simulink model "Tram_control_scheme"  (R2021a)
settings: Solver=VariableStepAuto  StartTime=0.0  StopTime=2000
values from neighbouring files (symbols this model uses):
  B = Tfriction/rated_speed_motor    (= 0.814101549937)    [Tram_script.m]
  d = 680e-3    (= 0.68)    [Tram_script.m]
  distance = [0,1,1.001,3,3.001,4,4.001,6,6.001,8,8.001,9,9.001,10]    [Tram_script.m]
  E = Van-Ra*Ian    (= 540)    [Tram_script.m]
  Ian = Pel_eq/Van    (= 155.555555556)    [Tram_script.m]
  Ien = 5    [Tram_script.m]
  J_eq = m_full_load*((speed_tram/3.6)^2)/(rated_speed_motor^2)    (= 85.9801387874)    [Tram_script.m]
  K = Tn/(Ian*Ien)    (= 1.06322065076)    [Tram_script.m]
  ki_a = par_regi.Ki    [Tram_script.m]
  ki_e = par_rege.Ki    [Tram_script.m]
  ki_O = par_reg_speed.Ki    [Tram_script.m]
  kp_a = par_regi.Kp    [Tram_script.m]
  kp_e = par_rege.Kp    [Tram_script.m]
  kp_O = par_reg_speed.Kp    [Tram_script.m]
  La = tau_a*Ra    (= 0.00385714285714)    [Tram_script.m]
  Le = Re*tau_e    (= 1.2)    [Tram_script.m]
  Ra = (1-efficiency)*Van/Ian    (= 0.385714285714)    [Tram_script.m]
  rated_speed_motor = Or*(2*pi)/60    (= 101.578162466)    [Tram_script.m]
  Re = Ven/Ien    (= 12)    [Tram_script.m]
  rho = 13/74    (= 0.175675675676)    [Tram_script.m]
  SatLow_T = -Tn*3    (= -2480.8481851)    [Tram_script.m]
  SatLow_Va = -Van    (= -600)    [Tram_script.m]
  SatLow_Ve = 0    [Tram_script.m]
  SatUp_T = Tn*3    (= 2480.8481851)    [Tram_script.m]
  SatUp_Va = Van    (= 600)    [Tram_script.m]
  SatUp_Ve = Ven*1.1    (= 66)    [Tram_script.m]
  speed_ref = [speed_tram/2,speed_tram/2, speed_tram,speed_tram,speed_tram,speed_tram,speed_max,speed_max,speed_tram,speed_tram,speed_tram,speed_tram,speed_tram/2,speed_tram/2]    [Tram_script.m]
  speed_weak = [0, speed_tram/4,speed_tram/2, speed_tram,speed_tram*1.5, speed_tram*1.8,speed_tram*1.9 speed_tram*2]    [Tram_script.m]
  T_weakening = [Tn, Tn, Tn, Tn, Tn/1.5, Tn/2, Tn/2.5, Tn/5]    [Tram_script.m]
  Tfriction = Tn/10    (= 82.6949395034)    [Tram_script.m]
  Ti_a = kp_a/ki_a    [Tram_script.m]
  Ti_e = kp_e/ki_e    [Tram_script.m]
  Ti_O = kp_O/ki_O    [Tram_script.m]
  Tn = Pmec_eq/rated_speed_motor    (= 826.949395034)    [Tram_script.m]
  Tslope = m_full_load*9.81*sin(theta)*d/2*rho    [Tram_script.m]
libraries: pid_lib x3, simulink x2, spspowerguiLib x1
settings Model: Creator=secch  LastModifiedBy=secch
settings SolverCC: AlgebraicLoopSolver=LineSearch
settings DebuggingCC: SFMachineParentedDataDiag=warning

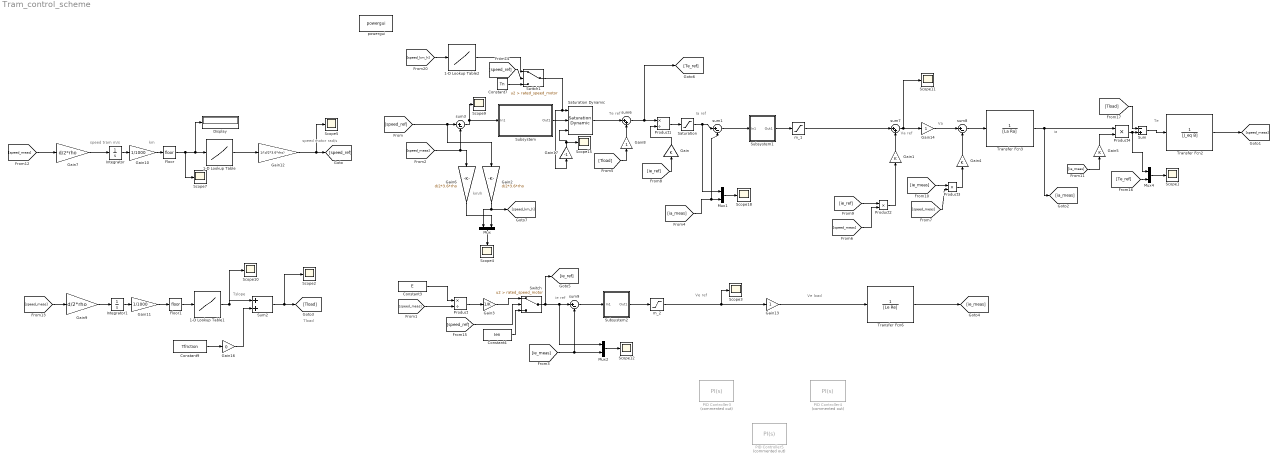
== system Tram_control_scheme ==
  note: km/h
  note: km
  note: speed tram
      | m/s
  note: speed motor
      | rad/s
  note: ia
  note: Va ref
  note: Ve load
  note: ie ref
  note: Te
  note: Ia ref
  note: Te ref
  note: Tload
  note: Tslope
  note: Ve ref
  note: Va
  1-D Lookup Table : Lookup_n-D  NumberOfTableDimensions=1  BreakpointsForDimension1=distance  Table=speed_ref  InternalRulePriority=Speed  RndMeth=Simplest  InputSameDT=on
  1-D Lookup Table1 : Lookup_n-D  NumberOfTableDimensions=1  BreakpointsForDimension1=distance  Table=Tslope  InternalRulePriority=Speed  RndMeth=Simplest  InputSameDT=on
  1-D Lookup Table2 : Lookup_n-D  NumberOfTableDimensions=1  BreakpointsForDimension1=speed_weak  Table=T_weakening  InternalRulePriority=Speed  RndMeth=Simplest  InputSameDT=on
  Constant3 : Constant  Value=E
  Constant4 : Constant  Value=Ien
  Constant7 : Constant  Value=Tn
  Constant9 : Constant  Value=Tfriction
  Display : Display
  Floor : Rounding
  Floor1 : Rounding
  Gain{,1,4..5} (4 alike) : Gain  Gain=K
  Gain10 : Gain  Gain=1/1000
  Gain11 : Gain  Gain=1/1000
  Gain12 : Gain  Gain=1/(d/2*3.6*rho)
  Gain13 : Gain
  Gain14 : Gain
  Gain16 : Gain  Gain=0
  Gain17 : Gain  Gain=-1
  Gain2 : Gain  Gain=d/2*3.6*rho
  Gain3 : Gain  Gain=1/K
  Gain6 : Gain  Gain=d/2*3.6*rho
  Gain7 : Gain  Gain=d/2*rho
  Gain8 : Gain
  Gain9 : Gain  Gain=d/2*rho
  Integrator : Integrator
  Integrator1 : Integrator
  Mux{,1..2,4} (4 alike) : Mux  Inputs=2
  PID Controller3 : pid_lib/PID Controller  Commented=on  Controller=PI  Form=Ideal  TimeDomain=Continuous-time  UseExternalTs=off  SampleTime=-1  IntegratorMethod=Forward Euler  FilterMethod=Forward Euler  ControllerParametersSource=internal  P=kp_O  I=ki_O  D=0  UseFilter=on  N=100  TunerSelectOption=Transfer Function Based (PID Tuner App)  InitialConditionSource=internal  InitialConditionForIntegrator=0  InitialConditionForFilter=0  DifferentiatorICPrevScaledInput=0  ExternalReset=none  TrackingMode=off  Kt=1  LimitOutput=on  SatLimitsSource=internal  UpperSaturationLimit=SatUp_T  LowerSaturationLimit=SatLow_T  LinearizeAsGain=on  AntiWindupMode=back-calculation  Kb=Ti_O  POutMin=[]  POutMax=[]  IOutMin=[]  IOutMax=[]  DOutMin=[]  DOutMax=[]  NOutMin=[]  NOutMax=[]  SumOutMin=[]  SumOutMax=[]  SaturationOutMin=[]  SaturationOutMax=[]  PParamMin=[]  PParamMax=[]  IParamMin=[]  IParamMax=[]  DParamMin=[]  DParamMax=[]  NParamMin=[]  NParamMax=[]  KbParamMin=[]  KbParamMax=[]  KtParamMin=[]  KtParamMax=[]  KbOutMin=[]  KbOutMax=[]  KtOutMin=[]  KtOutMax=[]  IntegratorOutMin=[]  IntegratorOutMax=[]  FilterOutMin=[]  FilterOutMax=[]  SumI1OutMin=[]  SumI1OutMax=[]  SumI2OutMin=[]  SumI2OutMax=[]  SumI3OutMin=[]  SumI3OutMax=[]  SumI4OutMin=[]  SumI4OutMax=[]  SumDOutMin=[]  SumDOutMax=[]  DifferentiatorOutMin=[]  DifferentiatorOutMax=[]  FilterDiffOutCoefMin=[]  FilterDiffOutCoefMax=[]  ReciprocalOutMin=[]  ReciprocalOutMax=[]  SumDenOutMin=[]  SumDenOutMax=[]  SumNumOutMin=[]  SumNumOutMax=[]  DivideOutMin=[]  DivideOutMax=[]  UdiffTsProdOutMin=[]  UdiffTsProdOutMax=[]  NTsProdOutMin=[]  NTsProdOutMax=[]  UintegralTsProdOutMin=[]  UintegralTsProdOutMax=[]  UngainTsProdOutMin=[]  UngainTsProdOutMax=[]  IntegratorContinuousStateAttributes=''  IntegratorStateMustResolveToSignalObject=off  IntegratorRTWStateStorageClass=Auto  FilterContinuousStateAttributes=''  FilterStateMustResolveToSignalObject=off  FilterRTWStateStorageClass=Auto  ParallelPVariant=Passthrough  IdealPVariant=InternalParameters  IVariant=InternalParameters  DVariant=Disabled  IntegratorVariant=Continuous  SatVariant=Enabled  AWVariant=BackCalculation  PCopyVariant=Disabled  TRVariant=Disabled  FdbkBlocksVariant=Forward  IdealPFdbkVariant=Disabled  SatFdbkVariant=Disabled  DerivativeFilterVariant=Disabled  NVariant=Disabled  NCopyVariant=Disabled_SignalSpec  FilterICVariant=Disabled  IntegratorICVariant=InternalICs  ExternalResetVariant=Disabled  TRSumVariant=Passthrough  SumFdbkVariant=Disabled  SumVariant=Sum_PI  TsampFilterVariant=InternalTs  TsampNgainVariant=Passthrough  TsampIntegralVariant=Passthrough  ExternalSaturationOutDataTypeStr=Inherit: Same as second input
  PID Controller4 : pid_lib/PID Controller  Commented=on  Controller=PI  Form=Ideal  TimeDomain=Continuous-time  UseExternalTs=off  SampleTime=-1  IntegratorMethod=Forward Euler  FilterMethod=Forward Euler  ControllerParametersSource=internal  P=kp_a  I=ki_a  D=0  UseFilter=on  N=100  TunerSelectOption=Transfer Function Based (PID Tuner App)  InitialConditionSource=internal  InitialConditionForIntegrator=0  InitialConditionForFilter=0  DifferentiatorICPrevScaledInput=0  ExternalReset=none  TrackingMode=off  Kt=1  LimitOutput=on  SatLimitsSource=internal  UpperSaturationLimit=SatUp_Va  LowerSaturationLimit=SatLow_Va  LinearizeAsGain=on  AntiWindupMode=back-calculation  Kb=Ti_a  POutMin=[]  POutMax=[]  IOutMin=[]  IOutMax=[]  DOutMin=[]  DOutMax=[]  NOutMin=[]  NOutMax=[]  SumOutMin=[]  SumOutMax=[]  SaturationOutMin=[]  SaturationOutMax=[]  PParamMin=[]  PParamMax=[]  IParamMin=[]  IParamMax=[]  DParamMin=[]  DParamMax=[]  NParamMin=[]  NParamMax=[]  KbParamMin=[]  KbParamMax=[]  KtParamMin=[]  KtParamMax=[]  KbOutMin=[]  KbOutMax=[]  KtOutMin=[]  KtOutMax=[]  IntegratorOutMin=[]  IntegratorOutMax=[]  FilterOutMin=[]  FilterOutMax=[]  SumI1OutMin=[]  SumI1OutMax=[]  SumI2OutMin=[]  SumI2OutMax=[]  SumI3OutMin=[]  SumI3OutMax=[]  SumI4OutMin=[]  SumI4OutMax=[]  SumDOutMin=[]  SumDOutMax=[]  DifferentiatorOutMin=[]  DifferentiatorOutMax=[]  FilterDiffOutCoefMin=[]  FilterDiffOutCoefMax=[]  ReciprocalOutMin=[]  ReciprocalOutMax=[]  SumDenOutMin=[]  SumDenOutMax=[]  SumNumOutMin=[]  SumNumOutMax=[]  DivideOutMin=[]  DivideOutMax=[]  UdiffTsProdOutMin=[]  UdiffTsProdOutMax=[]  NTsProdOutMin=[]  NTsProdOutMax=[]  UintegralTsProdOutMin=[]  UintegralTsProdOutMax=[]  UngainTsProdOutMin=[]  UngainTsProdOutMax=[]  IntegratorContinuousStateAttributes=''  IntegratorStateMustResolveToSignalObject=off  IntegratorRTWStateStorageClass=Auto  FilterContinuousStateAttributes=''  FilterStateMustResolveToSignalObject=off  FilterRTWStateStorageClass=Auto  ParallelPVariant=Passthrough  IdealPVariant=InternalParameters  IVariant=InternalParameters  DVariant=Disabled  IntegratorVariant=Continuous  SatVariant=Enabled  AWVariant=BackCalculation  PCopyVariant=Disabled  TRVariant=Disabled  FdbkBlocksVariant=Forward  IdealPFdbkVariant=Disabled  SatFdbkVariant=Disabled  DerivativeFilterVariant=Disabled  NVariant=Disabled  NCopyVariant=Disabled_SignalSpec  FilterICVariant=Disabled  IntegratorICVariant=InternalICs  ExternalResetVariant=Disabled  TRSumVariant=Passthrough  SumFdbkVariant=Disabled  SumVariant=Sum_PI  TsampFilterVariant=InternalTs  TsampNgainVariant=Passthrough  TsampIntegralVariant=Passthrough  ExternalSaturationOutDataTypeStr=Inherit: Same as second input
  PID Controller5 : pid_lib/PID Controller  Commented=on  Controller=PI  Form=Ideal  TimeDomain=Continuous-time  UseExternalTs=off  SampleTime=-1  IntegratorMethod=Forward Euler  FilterMethod=Forward Euler  ControllerParametersSource=internal  P=kp_e  I=ki_e  D=0  UseFilter=on  N=100  TunerSelectOption=Transfer Function Based (PID Tuner App)  InitialConditionSource=internal  InitialConditionForIntegrator=0  InitialConditionForFilter=0  DifferentiatorICPrevScaledInput=0  ExternalReset=none  TrackingMode=off  Kt=1  LimitOutput=on  SatLimitsSource=internal  UpperSaturationLimit=SatUp_Ve  LowerSaturationLimit=SatLow_Ve  LinearizeAsGain=on  AntiWindupMode=back-calculation  Kb=Ti_e  POutMin=[]  POutMax=[]  IOutMin=[]  IOutMax=[]  DOutMin=[]  DOutMax=[]  NOutMin=[]  NOutMax=[]  SumOutMin=[]  SumOutMax=[]  SaturationOutMin=[]  SaturationOutMax=[]  PParamMin=[]  PParamMax=[]  IParamMin=[]  IParamMax=[]  DParamMin=[]  DParamMax=[]  NParamMin=[]  NParamMax=[]  KbParamMin=[]  KbParamMax=[]  KtParamMin=[]  KtParamMax=[]  KbOutMin=[]  KbOutMax=[]  KtOutMin=[]  KtOutMax=[]  IntegratorOutMin=[]  IntegratorOutMax=[]  FilterOutMin=[]  FilterOutMax=[]  SumI1OutMin=[]  SumI1OutMax=[]  SumI2OutMin=[]  SumI2OutMax=[]  SumI3OutMin=[]  SumI3OutMax=[]  SumI4OutMin=[]  SumI4OutMax=[]  SumDOutMin=[]  SumDOutMax=[]  DifferentiatorOutMin=[]  DifferentiatorOutMax=[]  FilterDiffOutCoefMin=[]  FilterDiffOutCoefMax=[]  ReciprocalOutMin=[]  ReciprocalOutMax=[]  SumDenOutMin=[]  SumDenOutMax=[]  SumNumOutMin=[]  SumNumOutMax=[]  DivideOutMin=[]  DivideOutMax=[]  UdiffTsProdOutMin=[]  UdiffTsProdOutMax=[]  NTsProdOutMin=[]  NTsProdOutMax=[]  UintegralTsProdOutMin=[]  UintegralTsProdOutMax=[]  UngainTsProdOutMin=[]  UngainTsProdOutMax=[]  IntegratorContinuousStateAttributes=''  IntegratorStateMustResolveToSignalObject=off  IntegratorRTWStateStorageClass=Auto  FilterContinuousStateAttributes=''  FilterStateMustResolveToSignalObject=off  FilterRTWStateStorageClass=Auto  ParallelPVariant=Passthrough  IdealPVariant=InternalParameters  IVariant=InternalParameters  DVariant=Disabled  IntegratorVariant=Continuous  SatVariant=Enabled  AWVariant=BackCalculation  PCopyVariant=Disabled  TRVariant=Disabled  FdbkBlocksVariant=Forward  IdealPFdbkVariant=Disabled  SatFdbkVariant=Disabled  DerivativeFilterVariant=Disabled  NVariant=Disabled  NCopyVariant=Disabled_SignalSpec  FilterICVariant=Disabled  IntegratorICVariant=InternalICs  ExternalResetVariant=Disabled  TRSumVariant=Passthrough  SumFdbkVariant=Disabled  SumVariant=Sum_PI  TsampFilterVariant=InternalTs  TsampNgainVariant=Passthrough  TsampIntegralVariant=Passthrough  ExternalSaturationOutDataTypeStr=Inherit: Same as second input
  Product : Product  Inputs=*/
  Product1 : Product  Inputs=*/
  Product2 : Product
  Product3 : Product
  Product4 : Product
  Saturation : Saturate  UpperLimit=Ian  LowerLimit=-Ian
  Saturation Dynamic : simulink/Discontinuities/Saturation Dynamic  OutMin=[]  OutMax=[]  OutDataTypeStr=Inherit: Same as second input  OutDataType=fixdt(1, 16)  OutScaling=2^-10  DoSatur=off
  Scope{1..5,7,9..12,15,18} (12 alike) : Scope
  Subsystem : Subsystem
  Subsystem1 : Subsystem
  Subsystem2 : Subsystem
  Sum : Sum  Inputs=-+
  Sum2 : Sum  Inputs=|++
  Switch : Switch  Criteria=u2 > Threshold  Threshold=rated_speed_motor
  Switch1 : Switch  Criteria=u2 > Threshold  Threshold=rated_speed_motor
  Transfer Fcn2 : TransferFcn  Denominator=[J_eq B]
  Transfer Fcn3 : TransferFcn  Denominator=[La Ra]
  Transfer Fcn6 : TransferFcn  Denominator=[Le Re]
  m_1 : Saturate  UpperLimit=SatUp_Va  LowerLimit=SatLow_Va
  m_2 : Saturate  UpperLimit=SatUp_Ve  LowerLimit=SatLow_Ve
  powergui : spspowerguiLib/powergui  Priority=1  SimulationMode=Continuous  SampleTime=50e-6  frequency=60  Iterations=50  frequencyindice=0  Pbase=100e6  ErrMax=1e-4  UnitsV=kV  UnitsW=MW  buscounter=0  FunctionMessages=off  echomessages=off  EnableUseOfTLC=off  CurrentSourceSwitches=off  DisableSnubberDevices=off  DisableRonSwitches=off  DisableVfSwitches=off  DisplayEquations=off  AutomaticDiscreteSolvers=off  SolverType=Tustin/Backward Euler (TBE)  Interpol=off  ExternalGateDelay=off  methode=off  Ts=100  x0status=blocks  SPID=on  SwTol=0  HookPort=off  NonlinearTolerance=1e-4  nMaxIteration=100  ContinueOnMaxIteration=off  RestoreLinks=warning  ResistiveCurrentMeasurement=off  Frange=[0:2:500]  Ylog=off  Xlog=on  ShowGrid=off  save=off  variable=ZData  structure=0  ZoomFFT=off  StartTime=0.0  cycles=1  DisplayStyle=1  fundamental=60  FreqAxis=off  MaxFrequency=1000  frequencyindicesteady=1  RmsSteady=1  display=off
  sum{1,3,8..9} (4 alike) : Sum  Inputs=|+-
  sum6 : Sum  Inputs=|++
  sum7 : Sum  Inputs=|++
  wires:
  sum3/1 -> Subsystem/1(In1), Scope9/1
  [speed_ref] -> Gain2/1, sum3/1
  Product1/1 -> Saturation/1
  sum8/1 -> Transfer Fcn3/1
  Transfer Fcn3/1 -> [ia_meas], Product4/1
  Product4/1 -> Mux4/1, Sum/2
  Constant3/1 -> Product/1
  Gain3/1 -> Switch/1
  Product/1 -> Gain3/1
  Constant4/1 -> Switch/3
  1-D Lookup Table1/1 -> Scope10/1, Sum2/1
  Constant9/1 -> Gain16/1
  [speed_meas] -> sum3/2, Gain6/1
  Transfer Fcn2/1 -> [speed_meas]
  [ie_ref] -> Gain/1
  [ia_meas] -> Mux1/2, sum1/2
  Product3/1 -> Gain4/1
  Sum2/1 -> Scope2/1, [Tload]
  [Tload] -> Gain8/1
  [ie_ref] -> Product2/1
  Product2/1 -> Gain1/1
  [speed_meas] -> Product2/2
  [speed_meas] -> Product3/2
  [ie_meas] -> Product3/1
  Switch/1 -> [ie_ref], Mux2/1, sum9/1
  [ie_meas] -> Mux2/2, sum9/2
  Gain13/1 -> Transfer Fcn6/1
  Transfer Fcn6/1 -> [ie_meas]
  sum7/1 -> Gain14/1, Scope11/1
  Gain14/1 -> sum8/1
  [ie_meas] -> Gain5/1
  Gain/1 -> Product1/2
  Gain1/1 -> sum7/2
  Gain4/1 -> sum8/2
  Gain5/1 -> Product4/2
  Gain7/1 -> Integrator/1
  Integrator/1 -> Gain10/1
  Floor/1 -> Scope7/1, 1-D Lookup Table/1, Display/1
  Floor1/1 -> 1-D Lookup Table1/1
  Integrator1/1 -> Gain11/1
  [speed_meas] -> Gain9/1
  Gain9/1 -> Integrator1/1
  sum6/1 -> [Te_ref], Product1/1
  Mux/1 -> Scope4/1
  Gain10/1 -> Floor/1
  [speed_meas] -> Product/2
  Gain11/1 -> Floor1/1
  [speed_ref] -> Switch/2
  Subsystem1/1(Out1) -> m_1/1
  sum1/1 -> Subsystem1/1(In1)
  Subsystem2/1(Out1) -> m_2/1
  sum9/1 -> Subsystem2/1(In1)
  Gain2/1 -> [speed_km_h], Mux/1
  Gain6/1 -> Mux/2
  [speed_meas] -> Gain7/1
  [speed_ref] -> Switch1/2
  Constant7/1 -> Switch1/3
  Gain17/1 -> Saturation Dynamic/3, Scope15/1
  Subsystem/1(Out1) -> Saturation Dynamic/2
  Saturation Dynamic/1 -> sum6/1
  m_1/1 -> sum7/1
  m_2/1 -> Gain13/1, Scope3/1
  Mux1/1 -> Scope18/1
  Mux2/1 -> Scope12/1
  Gain12/1 -> Scope5/1, [speed_ref]
  1-D Lookup Table/1 -> Gain12/1
  Mux4/1 -> Scope1/1
  [Te_ref] -> Mux4/2
  Gain8/1 -> sum6/2
  Sum/1 -> Transfer Fcn2/1
  [Tload] -> Sum/1
  Gain16/1 -> Sum2/2
  Saturation/1 -> Mux1/1, sum1/1
  1-D Lookup Table2/1 -> Switch1/1
  Switch1/1 -> Gain17/1, Saturation Dynamic/1
  [speed_km_h] -> 1-D Lookup Table2/1

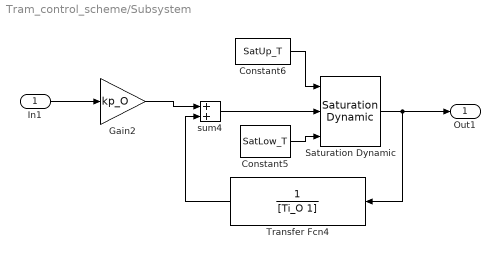
== system Tram_control_scheme/Subsystem ==
  In1 : Inport
  Constant5 : Constant  Value=SatLow_T
  Constant6 : Constant  Value=SatUp_T
  Gain2 : Gain  Gain=kp_O
  Saturation Dynamic : simulink/Discontinuities/Saturation Dynamic  OutMin=[]  OutMax=[]  OutDataTypeStr=Inherit: Same as second input  OutDataType=fixdt(1, 16)  OutScaling=2^-10  DoSatur=off
  Transfer Fcn4 : TransferFcn  Denominator=[Ti_O 1]
  sum4 : Sum
  Out1 : Outport
  wires:
  Transfer Fcn4/1 -> sum4/2
  Constant5/1 -> Saturation Dynamic/3
  Saturation Dynamic/1 -> Out1/1, Transfer Fcn4/1
  Constant6/1 -> Saturation Dynamic/1
  In1/1 -> Gain2/1
  sum4/1 -> Saturation Dynamic/2
  Gain2/1 -> sum4/1

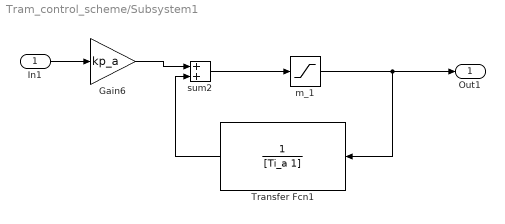
== system Tram_control_scheme/Subsystem1 ==
  In1 : Inport
  Gain6 : Gain  Gain=kp_a
  Transfer Fcn1 : TransferFcn  Denominator=[Ti_a 1]
  m_1 : Saturate  UpperLimit=SatUp_Va  LowerLimit=SatLow_Va
  sum2 : Sum
  Out1 : Outport
  wires:
  m_1/1 -> Out1/1, Transfer Fcn1/1
  In1/1 -> Gain6/1
  Transfer Fcn1/1 -> sum2/2
  Gain6/1 -> sum2/1
  sum2/1 -> m_1/1

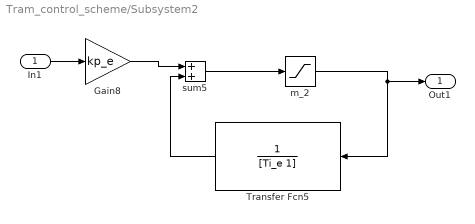
== system Tram_control_scheme/Subsystem2 ==
  In1 : Inport
  Gain8 : Gain  Gain=kp_e
  Transfer Fcn5 : TransferFcn  Denominator=[Ti_e 1]
  m_2 : Saturate  UpperLimit=SatUp_Ve  LowerLimit=SatLow_Ve
  sum5 : Sum
  Out1 : Outport
  wires:
  Transfer Fcn5/1 -> sum5/2
  In1/1 -> Gain8/1
  m_2/1 -> Out1/1, Transfer Fcn5/1
  Gain8/1 -> sum5/1
  sum5/1 -> m_2/1
